simulink model "three_ringnetwork_with_control"  (R2016a)
settings: Solver=VariableStepAuto  StartTime=0.0  StopTime=0.2  RelTol=1e-3
undefined symbols (not defined in the file): vc0d
libraries: simulink x18, powerlib_meascontrol x3
(part 3 of 3)

== matlab function three_ringnetwork_with_control/Init ==
  data: E0 output; E1 output; E2 output; E3 output; E4 output; U0 output; U1 output; U2 output; U3 output; U4 output; R1t0 output; R1t1 output; R1t2 output; R1t3 output; R1t4 output; R2t0 output; R2t1 output; R2t2 output; R2t3 output; R2t4 output; C0 output; C1 output; C2 output; C3 output; C4 output; L0 output; L1 output; L2 output; L3 output; L4 output; Lt0 output; Lt1 output; Lt2 output; Lt3 output; Lt4 output; Rab output; Lab output; Rac output; Lac output; il0d output; il1d output; il2d output; il3d output; il4d output; vc0ss output; vc1ss output; vc2ss output; vc3ss output; vc4ss output; ilt0ss output; ilt1ss output; ilt2ss output; ilt3ss output; ilt4ss output; iabss output; iacss output; Rab input; Rac input; E0 input; E1 input; Eb input; Ec input; m0 input
function [E0,E1,E2,E3,E4,U0,U1,U2,U3,U4,R1t0,R1t1,R1t2,R1t3,R1t4,R2t0,R2t1,R2t2,R2t3,R2t4,C0,C1,C2,C3,C4,L0,L1,L2,L3,L4,Lt0,Lt1,Lt2,Lt3,Lt4,Rab,Lab,Rac,Lac,il0d,il1d,il2d,il3d,il4d,vc0ss,vc1ss,vc2ss,vc3ss,vc4ss,ilt0ss,ilt1ss,ilt2ss,ilt3ss,ilt4ss,iabss,iacss]= fcn(Rab,Rac,E0,E1,Eb,Ec,m0)

%Rab=1000;
Lab=16e-3;
%Rac=1000;
Lac=16e-3;
e=1;
%E0=18;%+m1*4;%*m0;
%E0=E1=E2;/home/y-sadanda/share
%E1=18;
E2=18+e*m0;
E3=18+e*m0;%+6*m0;%+m1*14;
E4=18+e*m0;%+5*m1;%*m4;
% Eb=18;
% Ec=18;
%vd=40;
vd=40;%+8*sin(90*t);
U0=1-(E0/vd);
U1=1-(E1/vd);
U2=1-(E2/vd);
U3=1-(E3/vd);
U4=1-(E4/vd);

Ub=1-(Eb/vd);
Uc=1-(Ec/vd);
L0=46e-3;%*m0 ;
%L0=L1=L2;
L1=46e-3;%*m1 ;
L2=46e-3;%*m2 ;radians/sec to hertz
L3=46e-3;%*m3;
L4=46e-3;%*m4;

C0=100e-6;%*m0 ;
%C0=C1=C2;
C1=100e-6;%*m1 ;
C2=100e-6;%*m2 ;
C3=100e-6;%*m3;
C4=100e-6;%*m4;
%freq= 1/sqrt(L0*C0);

R1t0=10;
%R1t0R1t1=R2t2;
R1t1=10 ;
R1t2=10 ;
R1t3=10;
R1t4=10;

R2t0=100;%+100*m0 ;
%R2t0=R2t1=R2t2;
R2t1=100;%+100*m0;%*m1 ;
R2t2=100;%*m2 ;
R2t3=100;%*m3;
R2t4=100;%*m4;

Lt0=16e-3;%300e-3-270e-3*m0 ;
%Lt0=lt1=lt2;
Lt1=16e-3;%+270e-3*m0 ;
Lt2=16e-3 ;
Lt3=16e-3;
Lt4=16e-3;

vcbss=Eb/(1-Ub);
vccss=Ec/(1-Uc);

vc0ss=E0/(1-U0);
vc1ss=E1/(1-U1);
vc2ss=E2/(1-U2);
vc3ss=E3/(1-U3);
vc4ss=E4/(1-U4);



%Ast0=1/(sqrt((1-w0^2)^2+(w0/(Rb*sqrt(Lb/Cb)))));

% il0d = E0/(R2t4*(1-U0)^2)+((1/R1t0)*((E0/(1-U0)^2)-(E1/((1-U1)*(1-U0)))))-((1/R1t4)*(-(E0/(1-U0)^2)+(E4/((1-U4)*(1-U0)))));
% il1d = E1/(R2t0*(1-U1)^2)+((1/R1t1)*((E1/(1-U1)^2)-(E2/((1-U2)*(1-U1)))))-((1/R1t0)*(-(E1/(1-U1)^2)+(E0/((1-U0)*(1-U1)))));
% il2d = E2/(R2t1*(1-U2)^2)+((1/R1t2)*((E2/(1-U2)^2)-(E3/((1-U3)*(1-U2)))))-((1/R1t1)*(-(E2/(1-U2)^2)+(E1/((1-U1)*(1-U2)))));
% il3d = E3/(R2t2*(1-U3)^2)+((1/R1t3)*((E3/(1-U3)^2)-(E4/((1-U4)*(1-U3)))))-((1/R1t2)*(-(E3/(1-U3)^2)+(E2/((1-U2)*(1-U3)))));
% il4d = E4/(R2t3*(1-U4)^2)+((1/R1t4)*((E4/(1-U4)^2)-(E0/((1-U0)*(1-U4)))))-((1/R1t3)*(-(E4/(1-U4)^2)+(E3/((1-U3)*(1-U4)))));
% 
il0d = E0/(R2t4*(1-U0)^2)-((1/R1t0)*((E0/(1-U0)^2)-(E1/((1-U1)*(1-U0)))))+((1/R1t4)*(-(E0/(1-U0)^2)+(E4/((1-U4)*(1-U0)))))+((1/Rab)*((E0/(1-U0)^2)-(Eb/(1-Ub)*(1-U0))));
il1d = E1/(R2t0*(1-U1)^2)-((1/R1t1)*((E1/(1-U1)^2)-(E2/((1-U2)*(1-U1)))))+((1/R1t0)*(-(E1/(1-U1)^2)+(E0/((1-U0)*(1-U1)))))+((1/Rac)*((E1/(1-U1)^2)-(Ec/(1-Uc)*(1-U1))));
il2d = E2/(R2t1*(1-U2)^2)-((1/R1t2)*((E2/(1-U2)^2)-(E3/((1-U3)*(1-U2)))))+((1/R1t1)*(-(E2/(1-U2)^2)+(E1/((1-U1)*(1-U2)))));
il3d = E3/(R2t2*(1-U3)^2)-((1/R1t3)*((E3/(1-U3)^2)-(E4/((1-U4)*(1-U3)))))+((1/R1t2)*(-(E3/(1-U3)^2)+(E2/((1-U2)*(1-U3)))));
il4d = E4/(R2t3*(1-U4)^2)-((1/R1t4)*((E4/(1-U4)^2)-(E0/((1-U0)*(1-U4)))))+((1/R1t3)*(-(E4/(1-U4)^2)+(E3/((1-U3)*(1-U4)))));






ilt0ss=(1/R1t0)*(vc0ss-vc1ss);
ilt1ss=(1/R1t1)*(vc1ss-vc2ss);
ilt2ss=(1/R1t2)*(vc2ss-vc3ss);
ilt3ss=(1/R1t3)*(vc3ss-vc4ss);
ilt4ss=(1/R1t4)*(vc4ss-vc0ss);

iabss=(1/Rab)*(vc0ss-vcbss);
iacss=(1/Rac)*(vc1ss-vccss);

== matlab function three_ringnetwork_with_control/Init1 ==
  data: E0 output; E1 output; E2 output; E3 output; E4 output; U0 output; U1 output; U2 output; U3 output; U4 output; R1t0 output; R1t1 output; R1t2 output; R1t3 output; R1t4 output; R2t0 output; R2t1 output; R2t2 output; R2t3 output; R2t4 output; C0 output; C1 output; C2 output; C3 output; C4 output; L0 output; L1 output; L2 output; L3 output; L4 output; Lt0 output; Lt1 output; Lt2 output; Lt3 output; Lt4 output; il0d output; il1d output; il2d output; il3d output; il4d output; vc0ss output; vc1ss output; vc2ss output; vc3ss output; vc4ss output; ilt0ss output; ilt1ss output; ilt2ss output; ilt3ss output; ilt4ss output; E0 input; Rab input; Ea0 input; m1 input
function [E0,E1,E2,E3,E4,U0,U1,U2,U3,U4,R1t0,R1t1,R1t2,R1t3,R1t4,R2t0,R2t1,R2t2,R2t3,R2t4,C0,C1,C2,C3,C4,L0,L1,L2,L3,L4,Lt0,Lt1,Lt2,Lt3,Lt4,il0d,il1d,il2d,il3d,il4d,vc0ss,vc1ss,vc2ss,vc3ss,vc4ss,ilt0ss,ilt1ss,ilt2ss,ilt3ss,ilt4ss]= fcn(E0,Rab,Ea0,m1)

d=1;
%E0=18;%+m1*4;%*m0;
%E0=E1=E2;/home/y-sadanda/share
E1=18+d*m1;
E2=18+d*m1;%+6*m1;
E3=18+d*m1;%+m1*14;
E4=18+d*m1;%+5*m0;%*m4;
%Ea0=18;
%Rab=1000;
%vd=40;
vd=40;%+8*sin(90*t);
U0=1-(E0/vd);
U1=1-(E1/vd);
U2=1-(E2/vd);
U3=1-(E3/vd);
U4=1-(E4/vd);
Ua0=1-(Ea0/vd);

L0=46e-3;%*m0 ;
%L0=L1=L2;
L1=46e-3;%*m1 ;
L2=46e-3;%*m2 ;radians/sec to hertz
L3=46e-3;%*m3;
L4=46e-3;%*m4;

C0=100e-6;%*m0 ;
%C0=C1=C2;
C1=100e-6;%*m1 ;
C2=100e-6;%*m2 ;
C3=100e-6;%*m3;
C4=100e-6;%*m4;
freq= 1/sqrt(L0*C0);

R1t0=10;
%R1t0R1t1=R2t2;
R1t1=10 ;
R1t2=10 ;
R1t3=10;
R1t4=10;

R2t0=100;%+100*m0 ;
%R2t0=R2t1=R2t2;
R2t1=100;%+100*m0;%*m1 ;
R2t2=100;%*m2 ;
R2t3=100;%*m3;
R2t4=100;%*m4;

Lt0=16e-3;%300e-3-270e-3*m0 ;
%Lt0=lt1=lt2;
Lt1=16e-3;%+270e-3*m0 ;
Lt2=16e-3 ;
Lt3=16e-3;
Lt4=16e-3;


vc0ss=E0/(1-U0);
vc1ss=E1/(1-U1);
vc2ss=E2/(1-U2);
vc3ss=E3/(1-U3);
vc4ss=E4/(1-U4);



%Ast0=1/(sqrt((1-w0^2)^2+(w0/(Rb*sqrt(Lb/Cb)))));

% il0d = E0/(R2t4*(1-U0)^2)+((1/R1t0)*((E0/(1-U0)^2)-(E1/((1-U1)*(1-U0)))))-((1/R1t4)*(-(E0/(1-U0)^2)+(E4/((1-U4)*(1-U0)))));
% il1d = E1/(R2t0*(1-U1)^2)+((1/R1t1)*((E1/(1-U1)^2)-(E2/((1-U2)*(1-U1)))))-((1/R1t0)*(-(E1/(1-U1)^2)+(E0/((1-U0)*(1-U1)))));
% il2d = E2/(R2t1*(1-U2)^2)+((1/R1t2)*((E2/(1-U2)^2)-(E3/((1-U3)*(1-U2)))))-((1/R1t1)*(-(E2/(1-U2)^2)+(E1/((1-U1)*(1-U2)))));
% il3d = E3/(R2t2*(1-U3)^2)+((1/R1t3)*((E3/(1-U3)^2)-(E4/((1-U4)*(1-U3)))))-((1/R1t2)*(-(E3/(1-U3)^2)+(E2/((1-U2)*(1-U3)))));
% il4d = E4/(R2t3*(1-U4)^2)+((1/R1t4)*((E4/(1-U4)^2)-(E0/((1-U0)*(1-U4)))))-((1/R1t3)*(-(E4/(1-U4)^2)+(E3/((1-U3)*(1-U4)))));
% 
il0d = E0/(R2t4*(1-U0)^2)-((1/R1t0)*((E0/(1-U0)^2)-(E1/((1-U1)*(1-U0)))))+((1/R1t4)*(-(E0/(1-U0)^2)+(E4/((1-U4)*(1-U0)))))-((1/Rab)*((E0/(1-U0)^2)-(Ea0/((1-Ua0)*(1-U0)))));
il1d = E1/(R2t0*(1-U1)^2)-((1/R1t1)*((E1/(1-U1)^2)-(E2/((1-U2)*(1-U1)))))+((1/R1t0)*(-(E1/(1-U1)^2)+(E0/((1-U0)*(1-U1)))));
il2d = E2/(R2t1*(1-U2)^2)-((1/R1t2)*((E2/(1-U2)^2)-(E3/((1-U3)*(1-U2)))))+((1/R1t1)*(-(E2/(1-U2)^2)+(E1/((1-U1)*(1-U2)))));
il3d = E3/(R2t2*(1-U3)^2)-((1/R1t3)*((E3/(1-U3)^2)-(E4/((1-U4)*(1-U3)))))+((1/R1t2)*(-(E3/(1-U3)^2)+(E2/((1-U2)*(1-U3)))));
il4d = E4/(R2t3*(1-U4)^2)-((1/R1t4)*((E4/(1-U4)^2)-(E0/((1-U0)*(1-U4)))))+((1/R1t3)*(-(E4/(1-U4)^2)+(E3/((1-U3)*(1-U4)))));




ilt0ss=(1/R1t0)*(vc0ss-vc1ss);
ilt1ss=(1/R1t1)*(vc1ss-vc2ss);
ilt2ss=(1/R1t2)*(vc2ss-vc3ss);
ilt3ss=(1/R1t3)*(vc3ss-vc4ss);
ilt4ss=(1/R1t4)*(vc4ss-vc0ss);

== matlab function three_ringnetwork_with_control/Init2 ==
  data: E0 output; E1 output; E2 output; E3 output; E4 output; U0 output; U1 output; U2 output; U3 output; U4 output; R1t0 output; R1t1 output; R1t2 output; R1t3 output; R1t4 output; R2t0 output; R2t1 output; R2t2 output; R2t3 output; R2t4 output; C0 output; C1 output; C2 output; C3 output; C4 output; L0 output; L1 output; L2 output; L3 output; L4 output; Lt0 output; Lt1 output; Lt2 output; Lt3 output; Lt4 output; il0d output; il1d output; il2d output; il3d output; il4d output; vc0ss output; vc1ss output; vc2ss output; vc3ss output; vc4ss output; ilt0ss output; ilt1ss output; ilt2ss output; ilt3ss output; ilt4ss output; E0 input; Ea1 input; Rac input; m2 input
function [E0,E1,E2,E3,E4,U0,U1,U2,U3,U4,R1t0,R1t1,R1t2,R1t3,R1t4,R2t0,R2t1,R2t2,R2t3,R2t4,C0,C1,C2,C3,C4,L0,L1,L2,L3,L4,Lt0,Lt1,Lt2,Lt3,Lt4,il0d,il1d,il2d,il3d,il4d,vc0ss,vc1ss,vc2ss,vc3ss,vc4ss,ilt0ss,ilt1ss,ilt2ss,ilt3ss,ilt4ss]= fcn(E0,Ea1,Rac,m2)
f=1;

%E0=18;%+m1*4;%*m0;
%E0=E1=E2;/home/y-sadanda/share
E1=18+f*m2;
E2=18+f*m2;%+m0*7;
E3=18+f*m2;%+m1*14;
E4=18+f*m2;%+m1*6;%*m4;

%Ea1=18;
%Rac=1000;

%vd=40;
vd=40;%+8*sin(90*t);
U0=1-(E0/vd);
U1=1-(E1/vd);
U2=1-(E2/vd);
U3=1-(E3/vd);
U4=1-(E4/vd);

Ua1=1-(Ea1/vd);
L0=46e-3;%*m0 ;
%L0=L1=L2;
L1=46e-3;%*m1 ;
L2=46e-3;%*m2 ;radians/sec to hertz
L3=46e-3;%*m3;
L4=46e-3;%*m4;

C0=100e-6;%*m0 ;
%C0=C1=C2;
C1=100e-6;%*m1 ;
C2=100e-6;%*m2 ;
C3=100e-6;%*m3;
C4=100e-6;%*m4;
%freq= 1/sqrt(L0*C0);

R1t0=10;
%R1t0R1t1=R2t2;
R1t1=10 ;
R1t2=10 ;
R1t3=10;
R1t4=10;

R2t0=100;%+100*m0 ;
%R2t0=R2t1=R2t2;
R2t1=100;%+100*m0;%*m1 ;
R2t2=100;%*m2 ;
R2t3=100;%*m3;
R2t4=100;%*m4;

Lt0=16e-3;%300e-3-270e-3*m0 ;
%Lt0=lt1=lt2;
Lt1=16e-3;%+270e-3*m0 ;
Lt2=16e-3 ;
Lt3=16e-3;
Lt4=16e-3;


vc0ss=E0/(1-U0);
vc1ss=E1/(1-U1);
vc2ss=E2/(1-U2);
vc3ss=E3/(1-U3);
vc4ss=E4/(1-U4);


%Ast0=1/(sqrt((1-w0^2)^2+(w0/(Rb*sqrt(Lb/Cb)))));

% il0d = E0/(R2t4*(1-U0)^2)+((1/R1t0)*((E0/(1-U0)^2)-(E1/((1-U1)*(1-U0)))))-((1/R1t4)*(-(E0/(1-U0)^2)+(E4/((1-U4)*(1-U0)))));
% il1d = E1/(R2t0*(1-U1)^2)+((1/R1t1)*((E1/(1-U1)^2)-(E2/((1-U2)*(1-U1)))))-((1/R1t0)*(-(E1/(1-U1)^2)+(E0/((1-U0)*(1-U1)))));
% il2d = E2/(R2t1*(1-U2)^2)+((1/R1t2)*((E2/(1-U2)^2)-(E3/((1-U3)*(1-U2)))))-((1/R1t1)*(-(E2/(1-U2)^2)+(E1/((1-U1)*(1-U2)))));
% il3d = E3/(R2t2*(1-U3)^2)+((1/R1t3)*((E3/(1-U3)^2)-(E4/((1-U4)*(1-U3)))))-((1/R1t2)*(-(E3/(1-U3)^2)+(E2/((1-U2)*(1-U3)))));
% il4d = E4/(R2t3*(1-U4)^2)+((1/R1t4)*((E4/(1-U4)^2)-(E0/((1-U0)*(1-U4)))))-((1/R1t3)*(-(E4/(1-U4)^2)+(E3/((1-U3)*(1-U4)))));
% 
il0d = E0/(R2t4*(1-U0)^2)-((1/R1t0)*((E0/(1-U0)^2)-(E1/((1-U1)*(1-U0)))))+((1/R1t4)*(-(E0/(1-U0)^2)+(E4/((1-U4)*(1-U0)))))-((1/Rac)*((E0/(1-U0)^2)-(Ea1/((1-Ua1)*(1-U0)))));
il1d = E1/(R2t0*(1-U1)^2)-((1/R1t1)*((E1/(1-U1)^2)-(E2/((1-U2)*(1-U1)))))+((1/R1t0)*(-(E1/(1-U1)^2)+(E0/((1-U0)*(1-U1)))));
il2d = E2/(R2t1*(1-U2)^2)-((1/R1t2)*((E2/(1-U2)^2)-(E3/((1-U3)*(1-U2)))))+((1/R1t1)*(-(E2/(1-U2)^2)+(E1/((1-U1)*(1-U2)))));
il3d = E3/(R2t2*(1-U3)^2)-((1/R1t3)*((E3/(1-U3)^2)-(E4/((1-U4)*(1-U3)))))+((1/R1t2)*(-(E3/(1-U3)^2)+(E2/((1-U2)*(1-U3)))));
il4d = E4/(R2t3*(1-U4)^2)-((1/R1t4)*((E4/(1-U4)^2)-(E0/((1-U0)*(1-U4)))))+((1/R1t3)*(-(E4/(1-U4)^2)+(E3/((1-U3)*(1-U4)))));





ilt0ss=(1/R1t0)*(vc0ss-vc1ss);
ilt1ss=(1/R1t1)*(vc1ss-vc2ss);
ilt2ss=(1/R1t2)*(vc2ss-vc3ss);
ilt3ss=(1/R1t3)*(vc3ss-vc4ss);
ilt4ss=(1/R1t4)*(vc4ss-vc0ss);

== matlab function three_ringnetwork_with_control/cont/Lilt0ddot ==
  data: ilt0d input; Lilt0ddot output; vc0d input; vc1d input; R1t0 input
function Lilt0ddot = fcn(ilt0d,vc0d,vc1d,R1t0)
Lilt0ddot= (vc0d-vc1d) -(R1t0*ilt0d);

== matlab function three_ringnetwork_with_control/cont/Lilt1ddot ==
  data: ilt1d input; vc1d input; Lilt1ddot output; vc2d input; R1t1 input
function Lilt1ddot = fcn(ilt1d,vc1d,vc2d,R1t1)
Lilt1ddot= (vc1d-vc2d) -(R1t1*ilt1d);

== matlab function three_ringnetwork_with_control/utt/ut1v ==
  data: E1 input; ut1v output; Rbeta input; il1d input; il1 input
function ut1v = fcn(E1,Rbeta,il1d,il1)
ut1v = E1 +(Rbeta*(il1-il1d));

== matlab function three_ringnetwork_with_control/utt/ut2v ==
  data: E2 input; ut2v output; Rgamma input; il2d input; il2 input
function ut2v = fcn(E2,Rgamma,il2d,il2)
ut2v = E2 +(Rgamma*(il2-il2d));

== matlab function three_ringnetwork_with_control/utt/ut3v ==
  data: E3 input; ut3v output; Rdelta input; il3d input; il3 input
function ut3v = fcn(E3,Rdelta,il3d,il3)
ut3v = E3 +(Rdelta*(il3-il3d));

== matlab function three_ringnetwork_with_control/utt/ut0v ==
  data: E0 input; ut0v output; Ralpha input; il0d input; il0 input
function ut0v = fcn(E0,Ralpha,il0d,il0)
ut0v = E0 +(Ralpha*(il0-il0d));

== matlab function three_ringnetwork_with_control/utt/ut4v ==
  data: E4 input; ut4v output; Reta input; il4d input; il4 input
function ut4v = fcn(E4,Reta,il4d,il4)
ut4v = E4 +(Reta*(il4-il4d));

== matlab function three_ringnetwork_with_control/cont/Lilt2ddot ==
  data: ilt2d input; vc2d input; Lilt2ddot output; vc3d input; R1t2 input

function Lilt2ddot = fcn(ilt2d,vc2d,vc3d,R1t2)
Lilt2ddot= (vc2d-vc3d) -(R1t2*ilt2d);

== matlab function three_ringnetwork_with_control/cont/Lilt3ddot ==
  data: ilt3d input; vc3d input; Lilt3ddot output; vc4d input; R1t3 input

function Lilt3ddot = fcn(ilt3d,vc3d,vc4d,R1t3)
Lilt3ddot= (vc3d-vc4d) -(R1t3*ilt3d);

== matlab function three_ringnetwork_with_control/cont/Lilt4ddot ==
  data: ilt4d input; vc4d input; Lilt4ddot output; vc0d input; R1t4 input

function Lilt4ddot = fcn(ilt4d,vc4d,vc0d,R1t4)
Lilt4ddot= (vc4d-vc0d) -(R1t4*ilt4d);

== matlab function three_ringnetwork_with_control/cont/cvc0ddot ==
  data: ut0 input; Cvc0ddot output; il0d input; ilt0d input; ilt4d input; vc0d input; R2t4 input; iab input
function Cvc0ddot = fcn(ut0,il0d,ilt0d,ilt4d,vc0d,R2t4,iab)
Cvc0ddot=(1-ut0)*il0d- ilt0d+ ilt4d-(vc0d/R2t4)-iab;

== matlab function three_ringnetwork_with_control/cont/cvc1ddot ==
  data: ut1 input; Cvc1ddot output; il1d input; ilt1d input; ilt0d input; vc1d input; R2t0 input; iac input
function Cvc1ddot = fcn(ut1,il1d,ilt1d,ilt0d,vc1d,R2t0,iac)
Cvc1ddot=(1-ut1)*il1d- ilt1d+ ilt0d-(vc1d/R2t0)-iac;

== matlab function three_ringnetwork_with_control/cont/cvc2ddot ==
  data: ut2 input; Cvc2ddot output; il2d input; ilt2d input; ilt1d input; vc2d input; R2t1 input
function Cvc2ddot = fcn(ut2,il2d,ilt2d,ilt1d,vc2d,R2t1)
Cvc2ddot=(1-ut2)*il2d- ilt2d+ ilt1d-(vc2d/R2t1);

== matlab function three_ringnetwork_with_control/cont/cvc3ddot ==
  data: ut3 input; Cvc3ddot output; il3d input; ilt3d input; ilt2d input; vc3d input; R2t2 input
function Cvc3ddot = fcn(ut3,il3d,ilt3d,ilt2d,vc3d,R2t2)
Cvc3ddot=(1-ut3)*il3d- ilt3d+ ilt2d-(vc3d/R2t2);

== matlab function three_ringnetwork_with_control/cont/cvc3ddot1 ==
  data: ut4 input; Cvc4ddot output; il4d input; ilt4d input; ilt3d input; vc4d input; R2t3 input
function Cvc4ddot = fcn(ut4,il4d,ilt4d,ilt3d,vc4d,R2t3)
Cvc4ddot=(1-ut4)*il4d- ilt4d+ ilt3d-(vc4d/R2t3);

== matlab function three_ringnetwork_with_control/cont/iab ==
  data: iab input; vc0 input; Labddot output; vcb input; Rab input

function Labddot = fcn(iab,vc0,vcb,Rab)
Labddot= (vc0-vcb) -(Rab*iab);

== matlab function three_ringnetwork_with_control/cont/iab1 ==
  data: iac input; vc1 input; Lacddot output; vcc input; Rac input

function Lacddot = fcn(iac,vc1,vcc,Rac)
Lacddot= (vc1-vcc) -(Rac*iac);

== matlab function three_ringnetwork_with_control/utt1/ut0v ==
  data: E0 input; ut0v output; Ralpha input; il0d input; il0 input
function ut0v = fcn(E0,Ralpha,il0d,il0)
ut0v = E0 +(Ralpha*(il0-il0d));

== matlab function three_ringnetwork_with_control/utt1/ut1v ==
  data: E1 input; ut1v output; Rbeta input; il1d input; il1 input
function ut1v = fcn(E1,Rbeta,il1d,il1)
ut1v = E1 +(Rbeta*(il1-il1d));

== matlab function three_ringnetwork_with_control/utt1/ut2v ==
  data: E2 input; ut2v output; Rgamma input; il2d input; il2 input
function ut2v = fcn(E2,Rgamma,il2d,il2)
ut2v = E2 +(Rgamma*(il2-il2d));

== matlab function three_ringnetwork_with_control/utt1/ut3v ==
  data: E3 input; ut3v output; Rdelta input; il3d input; il3 input
function ut3v = fcn(E3,Rdelta,il3d,il3)
ut3v = E3 +(Rdelta*(il3-il3d));

== matlab function three_ringnetwork_with_control/utt1/ut4v ==
  data: E4 input; ut4v output; Reta input; il4d input; il4 input
function ut4v = fcn(E4,Reta,il4d,il4)
ut4v = E4 +(Reta*(il4-il4d));

== matlab function three_ringnetwork_with_control/cont1/Lilt0ddot ==
  data: ilt0d input; Lilt0ddot output; vc0d input; vc1d input; R1t0 input
function Lilt0ddot = fcn(ilt0d,vc0d,vc1d,R1t0)
Lilt0ddot= (vc0d-vc1d) -(R1t0*ilt0d);

== matlab function three_ringnetwork_with_control/cont1/Lilt1ddot ==
  data: ilt1d input; vc1d input; Lilt1ddot output; vc2d input; R1t1 input
function Lilt1ddot = fcn(ilt1d,vc1d,vc2d,R1t1)
Lilt1ddot= (vc1d-vc2d) -(R1t1*ilt1d);

== matlab function three_ringnetwork_with_control/cont1/Lilt2ddot ==
  data: ilt2d input; vc2d input; Lilt2ddot output; vc3d input; R1t2 input

function Lilt2ddot = fcn(ilt2d,vc2d,vc3d,R1t2)
Lilt2ddot= (vc2d-vc3d) -(R1t2*ilt2d);

== matlab function three_ringnetwork_with_control/cont1/Lilt3ddot ==
  data: ilt3d input; vc3d input; Lilt3ddot output; vc4d input; R1t3 input

function Lilt3ddot = fcn(ilt3d,vc3d,vc4d,R1t3)
Lilt3ddot= (vc3d-vc4d) -(R1t3*ilt3d);

== matlab function three_ringnetwork_with_control/cont1/Lilt4ddot ==
  data: ilt4d input; vc4d input; Lilt4ddot output; vc0d input; R1t4 input

function Lilt4ddot = fcn(ilt4d,vc4d,vc0d,R1t4)
Lilt4ddot= (vc4d-vc0d) -(R1t4*ilt4d);

== matlab function three_ringnetwork_with_control/cont1/cvc0ddot ==
  data: ut0 input; Cvc0ddot output; il0d input; ilt0d input; ilt4d input; vc0d input; R2t4 input; iabd input
function Cvc0ddot = fcn(ut0,il0d,ilt0d,ilt4d,vc0d,R2t4,iabd)
Cvc0ddot=(1-ut0)*il0d- ilt0d+ ilt4d-(vc0d/R2t4)+iabd;

== matlab function three_ringnetwork_with_control/cont1/cvc1ddot ==
  data: ut1 input; Cvc1ddot output; il1d input; ilt1d input; ilt0d input; vc1d input; R2t0 input
function Cvc1ddot = fcn(ut1,il1d,ilt1d,ilt0d,vc1d,R2t0)
Cvc1ddot=(1-ut1)*il1d- ilt1d+ ilt0d-(vc1d/R2t0);

== matlab function three_ringnetwork_with_control/cont1/cvc2ddot ==
  data: ut2 input; Cvc2ddot output; il2d input; ilt2d input; ilt1d input; vc2d input; R2t1 input
function Cvc2ddot = fcn(ut2,il2d,ilt2d,ilt1d,vc2d,R2t1)
Cvc2ddot=(1-ut2)*il2d- ilt2d+ ilt1d-(vc2d/R2t1);

== matlab function three_ringnetwork_with_control/cont1/cvc3ddot ==
  data: ut3 input; Cvc3ddot output; il3d input; ilt3d input; ilt2d input; vc3d input; R2t2 input
function Cvc3ddot = fcn(ut3,il3d,ilt3d,ilt2d,vc3d,R2t2)
Cvc3ddot=(1-ut3)*il3d- ilt3d+ ilt2d-(vc3d/R2t2);

== matlab function three_ringnetwork_with_control/cont1/cvc3ddot1 ==
  data: ut4 input; Cvc4ddot output; il4d input; ilt4d input; ilt3d input; vc4d input; R2t3 input
function Cvc4ddot = fcn(ut4,il4d,ilt4d,ilt3d,vc4d,R2t3)
Cvc4ddot=(1-ut4)*il4d- ilt4d+ ilt3d-(vc4d/R2t3);

== matlab function three_ringnetwork_with_control/cont2/Lilt0ddot ==
  data: ilt0d input; Lilt0ddot output; vc0d input; vc1d input; R1t0 input
function Lilt0ddot = fcn(ilt0d,vc0d,vc1d,R1t0)
Lilt0ddot= (vc0d-vc1d) -(R1t0*ilt0d);

== matlab function three_ringnetwork_with_control/cont2/Lilt1ddot ==
  data: ilt1d input; vc1d input; Lilt1ddot output; vc2d input; R1t1 input
function Lilt1ddot = fcn(ilt1d,vc1d,vc2d,R1t1)
Lilt1ddot= (vc1d-vc2d) -(R1t1*ilt1d);

== matlab function three_ringnetwork_with_control/cont2/Lilt2ddot ==
  data: ilt2d input; vc2d input; Lilt2ddot output; vc3d input; R1t2 input

function Lilt2ddot = fcn(ilt2d,vc2d,vc3d,R1t2)
Lilt2ddot= (vc2d-vc3d) -(R1t2*ilt2d);

== matlab function three_ringnetwork_with_control/cont2/Lilt3ddot ==
  data: ilt3d input; vc3d input; Lilt3ddot output; vc4d input; R1t3 input

function Lilt3ddot = fcn(ilt3d,vc3d,vc4d,R1t3)
Lilt3ddot= (vc3d-vc4d) -(R1t3*ilt3d);

== matlab function three_ringnetwork_with_control/cont2/Lilt4ddot ==
  data: ilt4d input; vc4d input; Lilt4ddot output; vc0d input; R1t4 input

function Lilt4ddot = fcn(ilt4d,vc4d,vc0d,R1t4)
Lilt4ddot= (vc4d-vc0d) -(R1t4*ilt4d);

== matlab function three_ringnetwork_with_control/cont2/cvc0ddot ==
  data: ut0 input; Cvc0ddot output; il0d input; ilt0d input; ilt4d input; vc0d input; R2t4 input; iacd input
function Cvc0ddot = fcn(ut0,il0d,ilt0d,ilt4d,vc0d,R2t4,iacd)
Cvc0ddot=(1-ut0)*il0d- ilt0d+ ilt4d-(vc0d/R2t4)+iacd;

== matlab function three_ringnetwork_with_control/cont2/cvc1ddot ==
  data: ut1 input; Cvc1ddot output; il1d input; ilt1d input; ilt0d input; vc1d input; R2t0 input
function Cvc1ddot = fcn(ut1,il1d,ilt1d,ilt0d,vc1d,R2t0)
Cvc1ddot=(1-ut1)*il1d- ilt1d+ ilt0d-(vc1d/R2t0);

== matlab function three_ringnetwork_with_control/cont2/cvc2ddot ==
  data: ut2 input; Cvc2ddot output; il2d input; ilt2d input; ilt1d input; vc2d input; R2t1 input
function Cvc2ddot = fcn(ut2,il2d,ilt2d,ilt1d,vc2d,R2t1)
Cvc2ddot=(1-ut2)*il2d- ilt2d+ ilt1d-(vc2d/R2t1);

== matlab function three_ringnetwork_with_control/cont2/cvc3ddot ==
  data: ut3 input; Cvc3ddot output; il3d input; ilt3d input; ilt2d input; vc3d input; R2t2 input
function Cvc3ddot = fcn(ut3,il3d,ilt3d,ilt2d,vc3d,R2t2)
Cvc3ddot=(1-ut3)*il3d- ilt3d+ ilt2d-(vc3d/R2t2);

== matlab function three_ringnetwork_with_control/cont2/cvc3ddot1 ==
  data: ut4 input; Cvc4ddot output; il4d input; ilt4d input; ilt3d input; vc4d input; R2t3 input
function Cvc4ddot = fcn(ut4,il4d,ilt4d,ilt3d,vc4d,R2t3)
Cvc4ddot=(1-ut4)*il4d- ilt4d+ ilt3d-(vc4d/R2t3);

== matlab function three_ringnetwork_with_control/utt2/ut0v ==
  data: E0 input; ut0v output; Ralpha input; il0d input; il0 input
function ut0v = fcn(E0,Ralpha,il0d,il0)
ut0v = E0 +(Ralpha*(il0-il0d));

== matlab function three_ringnetwork_with_control/utt2/ut1v ==
  data: E1 input; ut1v output; Rbeta input; il1d input; il1 input
function ut1v = fcn(E1,Rbeta,il1d,il1)
ut1v = E1 +(Rbeta*(il1-il1d));

== matlab function three_ringnetwork_with_control/utt2/ut2v ==
  data: E2 input; ut2v output; Rgamma input; il2d input; il2 input
function ut2v = fcn(E2,Rgamma,il2d,il2)
ut2v = E2 +(Rgamma*(il2-il2d));

== matlab function three_ringnetwork_with_control/utt2/ut3v ==
  data: E3 input; ut3v output; Rdelta input; il3d input; il3 input
function ut3v = fcn(E3,Rdelta,il3d,il3)
ut3v = E3 +(Rdelta*(il3-il3d));

== matlab function three_ringnetwork_with_control/utt2/ut4v ==
  data: E4 input; ut4v output; Reta input; il4d input; il4 input
function ut4v = fcn(E4,Reta,il4d,il4)
ut4v = E4 +(Reta*(il4-il4d));

== matlab function three_ringnetwork_with_control/MATLAB Function ==
  data: Ea0 output; Ea1 output; Eb0 output; Ec0 output; Rab output; Rac output; m0 input; m1 input; m2 input
function [Ea0,Ea1,Eb0,Ec0,Rab,Rac] = fcn(m0,m1,m2)
%#codegen
d=1;
e=1;
f=1;
Ea0=18+e*m0;
Ea1=18+e*m0;%+m3;
Eb0=18+d*m1;
Ec0=18+f*m2;
Rab=500;
Rac=500;
